simulink model "GyroNoiseGenerate"  (Simulink 8.3)
settings: Solver=ode3  SolverMode=SingleTasking  StartTime=0.0  StopTime=" 6*3600"  FixedStep=0.004  RelTol=1e-3
settings Model: Creator=Administrator  LastModifiedBy=dell  CovMetricSettings=dwe  CovHtmlReporting=off  covSaveCumulativeToWorkspaceVar=off  CovSaveSingleToWorkspaceVar=off  CovExternalEMLEnable=on  CovSFcnEnable=on
settings DataIOCC: LimitDataPoints=off  SaveFormat=StructureWithTime  SignalLoggingSaveFormat=Dataset
settings DebuggingCC: UnderspecifiedInitializationDetection=Simplified  MergeDetectMultiDrivingBlocksExec=error  SolverPrmCheckMsg=none  FrameProcessingCompatibilityMsg=error  StateNameClashWarn=none  SFUnexpectedBacktrackingDiag=error  SFNoUnconditionalDefaultTransitionDiag=error
settings HardwareCC: ProdBitPerPointer=64  ProdLargestAtomicFloat=Float  ProdIntDivRoundTo=Zero  ProdEndianess=LittleEndian  ProdHWDeviceType=Specified
settings ModelReferenceCC: PropagateSignalLabelsOutOfModel=on
settings GRTTargetCC: TargetLangStandard=C99 (ISO)  GeneratePreprocessorConditionals=Use local settings  CombineOutputUpdateFcns=on  GRTInterface=off

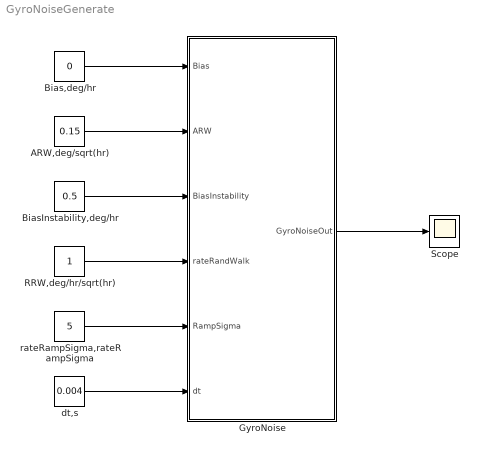
== system GyroNoiseGenerate ==
  ARW,deg/sqrt(hr) : Constant  Value=0.15
  Bias,deg/hr : Constant  Value=0
  BiasInstability,deg/hr : Constant  Value=0.5
  GyroNoise : MATLAB Function  TreatAsAtomicUnit=on
      settings: PermitHierarchicalResolution=ParametersOnly
  RRW,deg/hr/sqrt(hr) : Constant
  Scope : Scope
      settings: TimeRange=auto  MaxDataPoints=5000  SaveToWorkspace=off  SaveName=ScopeData  YMin=-0.03422  YMax=0.0509  SampleTime=-1
  dt,s : Constant  Value=0.004
  rateRampSigma,rateRampSigma : Constant  Value=5
  wires:
  Bias,deg/hr/1 -> GyroNoise/1(Bias)
  BiasInstability,deg/hr/1 -> GyroNoise/3(BiasInstability)
  ARW,deg/sqrt(hr)/1 -> GyroNoise/2(ARW)
  dt,s/1 -> GyroNoise/6(dt)
  GyroNoise/1(GyroNoiseOut) -> Scope/1
  RRW,deg/hr/sqrt(hr)/1 -> GyroNoise/4(rateRandWalk)
  rateRampSigma,rateRampSigma/1 -> GyroNoise/5(RampSigma)

== matlab function GyroNoise ==
  data: Bias input double; ARW input double; GyroNoiseOut output double; BiasInstability input double; rateRandWalk input double; RampSigma input double; dt input double
function GyroNoiseOut  = fcn(Bias,ARW,BiasInstability,rateRandWalk,RampSigma,dt)
%#codegen

%输入 零偏 deg/hr,零偏不稳定性deg/hr,角度随机游走deg/sqrt(hr),采样时间间隔
persistent  biasNoiseDot RRNoiseDotDot_per RRWNoiseDotDot_per


if isempty(biasNoiseDot)
    biasNoiseDot = 0;
end
if isempty(RRNoiseDotDot_per)
    RRNoiseDotDot_per = 0;
end
if isempty(RRWNoiseDotDot_per)
    RRWNoiseDotDot_per = 0;
end



SigmaRW = ARW/60/sqrt(dt); % Converted sigma to deg/s or m/s^2
RWNoiseDot = SigmaRW*randn(1,1); % WGN noise signal

% Bias Instability is generated with either flicker (pink) noise or
% approximated by a First Order Gauss Markov signal with appropriate
% strength and correlation time. The input coefficient was in deg/hr or
% m/s/hr, so we need to convert to the units of our output signal (deg/s or
% m/s^2).
SigmaBias = BiasInstability/3600; % Converted to deg/s or m/s^2

% Direct Flicker Noise Method

    % FOGM Approximation Method
    Tbias = 0.0119*3600;
    tc = Tbias/1.89;
    Q = SigmaBias;
    Qd = Q^2*(1 - exp(-2*dt/tc));
    phi = exp(-dt/tc);
    

    
    BiasInstabilityOut =  phi*biasNoiseDot + sqrt(Qd)*randn;
   
    biasNoiseDot = BiasInstabilityOut;
    
    
    
% Rate Random Walk refers to a random walk that is manifested in the rate
% output (deg/s or m/s^2). This means the random walk came from WGN found
% in the derrivative of the rate output. Namely in a signal that is the
% derrivative of our desired output signal. To simulate RRW, we will then
% apply WGN to a signal and integrate it once to produce our desired output
% signal. Same unit conversion applies here as we take in deg/hr/sqrt(hr)
% or m/s/hr/sqrt(hr) and convert to deg/s or m/s^2



    SigmaRRW = rateRandWalk/(3600*60)*sqrt(dt)/dt; % [deg/s^2] or [m/s/s^2]
    RRWNoiseDotDo = SigmaRRW*randn(1,1);
    RRWNoiseDotOut = RRWNoiseDotDot_per+RRWNoiseDotDo*dt; % In deg/s or m/s/s
    RRWNoiseDotDot_per=RRWNoiseDotOut;
    
    
    % Rate Ramp [deg/hr/hr]
    R = RampSigma/(3600*3600); % [deg/s/s]
    RRNoiseDotDot = ones(1,1)*R;   
    RRNoiseDotOut = RRNoiseDotDot_per+RRNoiseDotDot*dt; % In deg/s or m/s/s
    RRNoiseDotDot_per=RRNoiseDotOut;

% Finally, the output signal in deg/s or m/s^2 is constructed by adding all
% noise sources since they are assumed to be independent. Note that
% IEEE-STD-952-1997 specifices Allan Variances add linearly, which is not
% contradicted by this sum since these are not variances but rather time
% domain signals.

GyroNoiseOut = Bias + RWNoiseDot + BiasInstabilityOut+RRWNoiseDotOut+RRNoiseDotOut;

end
